simulink model "LQ_observer_simulation"  (R2019a)
settings: Solver=VariableStepAuto  StartTime=0.0  StopTime=24  RelTol=1e-3
values from neighbouring files (symbols this model uses):
  A = modeld.a    [LQR_initialization.m]    (also in LQ_observer_initialization.m; MPC_initialization.m = sysd.a; MagnetoShield_LQ_Initialization.m; MagnetoShield_PolePlacement_Initialization.m)
  B = modeld.b    [LQR_initialization.m]    (also in LQ_observer_initialization.m; MPC_initialization.m = sysd.b; MagnetoShield_LQ_Initialization.m; MagnetoShield_PolePlacement_Initialization.m)
  C = [1 0 0;0 0 1]    [LQR_initialization.m]    (also in LQ_observer_initialization.m = [1 0 0]; MPC_initialization.m = [1 0 0]; MagnetoShield_LQ_Initialization.m; MagnetoShield_PolePlacement_Initialization.m = [1 0 0])
  i0 = 0.00301720799779    [MagnetoShield_Alternative_model.mat]    (also in MagnetoShield_Models_Greybox_SS model.mat = 0.0219057293333)
  K = dlqr(Ai,Bi,Qlq,Rlq)    [LQR_initialization.m]    (also in LQ_observer_initialization.m; MagnetoShield_LQ_Initialization.m; MagnetoShield_PolePlacement_Initialization.m = [0 0 0 1]*inv([Bi Ai*Bi Ai^2*Bi Ai^3*Bi])*phy)
  L = phy*inv([C; C*A; C*A^2])*[0 0 1]'    [LQ_observer_initialization.m]    (also in MagnetoShield_PolePlacement_Initialization.m)
  Ts = 0.001    [LQR_initialization.m]    (also in LQ_observer_initialization.m = 0.002; MPC_initialization.m; MagnetoShield_LQ_Initialization.m = 0.0015; MagnetoShield_PolePlacement_Initialization.m = 0.0015)
  u0 = 0.633613679536    [MagnetoShield_Alternative_model.mat]    (also in MagnetoShield_Models_Greybox_SS model.mat = 4.62338933333)
  y0 = 0.012    [MagnetoShield_Alternative_model.mat]    (also in MagnetoShield_Models_Greybox_SS model.mat = 0.0143094466667)
undefined symbols (not defined in the file or in its folder): DiscIntNeverNeededParam
libraries: simulink x2
settings Model: Creator=jakub  LastModifiedBy=jakub
settings SolverCC: AlgebraicLoopSolver=LineSearch

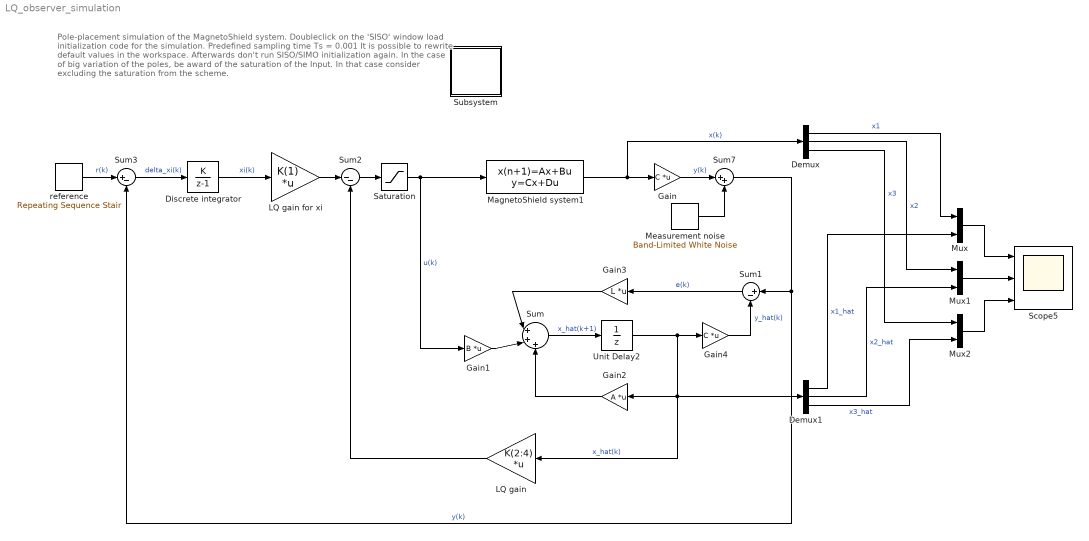
== system LQ_observer_simulation ==
  note: Pole-placement simulation of the  MagnetoShield system.
      | Doubleclick on the 'SISO' window load initialization code for the simulation.
      | Predefined sampling time Ts = 0.001
      | It is possible to rewrite default values in the workspace.  Afterwards don't run SISO/SIMO
      | initialization again.
      |
      | In the case of big variation of the poles, be award of the saturation of the Input. In that case
      | consider excluding the saturation from the scheme.
  Demux : Demux  Outputs=3
  Demux1 : Demux  Outputs=3
  Discrete integrator : DiscreteIntegrator  IntegratorMethod=Accumulation: Forward Euler  SampleTime=Ts  LimitOutput=on  UpperSaturationLimit=1  LowerSaturationLimit=-1  ICPrevOutput=DiscIntNeverNeededParam  ICPrevScaledInput=DiscIntNeverNeededParam
  Gain : Gain  Gain=C  Multiplication=Matrix(K*u)
  Gain1 : Gain  Gain=B  Multiplication=Matrix(K*u)
  Gain2 : Gain  Gain=A  Multiplication=Matrix(K*u)
  Gain3 : Gain  Gain=L  Multiplication=Matrix(K*u)
  Gain4 : Gain  Gain=C  Multiplication=Matrix(K*u)
  LQ gain : Gain  Gain=K(2:4)  Multiplication=Matrix(K*u)
  LQ gain for xi : Gain  Gain=K(1)  Multiplication=Matrix(K*u)
  MagnetoShield system1 : DiscreteStateSpace  A=A  B=B  C=[1 0 0;0 1 0;0 0 1]  D=[0;0;0]  InitialCondition=[0.017-y0;0;0-i0]  SampleTime=Ts
  Measurement noise : simulink/Sources/Band-Limited White Noise  Cov=[(2*10^(-8))^2]  Ts=2*Ts  seed=[23341]
  Mux : Mux  Inputs=2
  Mux1 : Mux  Inputs=2
  Mux2 : Mux  Inputs=2
  Saturation : Saturate  UpperLimit=12-u0  LowerLimit=0-u0
  Scope5 : Scope  NumInputPorts=3
  Subsystem : Subsystem
      settings: OpenFcn=|
      | clear;close all;clc;
      | load '../../../matlab/examples/MagnetoShield/MagnetoShield_Models_Greybox_SS';
      | %% MagnetoShield - Pole-placement simulation and control initialization for Simulink
      | Ts = 0.001;                   % Sampling of the Simulink simulation
      | 
      | % Matrices extraction from model
      | modeld=c2d(model,Ts);           % Discretized linear state-space model
      | A = modeld.a;                   % Extract A
      | B = modeld.b;                   % Extract B
      | C = [1 0 0];                   % Position is measured for integrator 'xi' computation
      | 
      | % Discrete augmented model with integrator state - unstable, unobservable
      | Ai = [1 -C;
      |       zeros(3,1) A];
      | Bi = [0;B];
      | 
      | % Observer gain L computation
      | polesL = [-0.003 0.0006715 -0.00003715]; % desired poles of observer
      | p = poly(polesL);                        % polynomial coeficients
      | I = eye(size(A));
      | phy = p(4)*I+p(3)*A+p(2)*A^2+A^3;
      | L = phy*inv([C; C*A; C*A^2])*[0 0 1]';   % Ackermann's formula for observer
      | 
      | % Pole-placement gain K for augmented system
      | polesK = [0.985 0.5353 0.826 0.9581];       % desired poles of the system
      | p = poly(polesK);                           % polynomial coeficients
      | I = eye(size(Ai));
      | phy = p(5)*I+p(4)*Ai+p(3)*Ai^2+p(2)*Ai^3+Ai^4;
      | K = [0 0 0 1]*inv([Bi Ai*Bi Ai^2*Bi Ai^3*Bi])*phy; % Ackermann's formula for gain K
      mask Display: disp('SISO')
  Sum : Sum  Inputs=|+++
  Sum1 : Sum  Inputs=|+-
  Sum2 : Sum  Inputs=|--
  Sum3 : Sum  Inputs=|+-
  Sum7 : Sum  Inputs=|++
  Unit Delay2 : UnitDelay  InitialCondition=[0.017-y0;0;0-i0]  SampleTime=-1  HasFrameUpgradeWarning=on
  reference : simulink/Sources/Repeating Sequence Stair  OutValues=[ones(1,2000)*(0.013-y0) ones(1,2000)*(0.016-y0) ones(1,2000)*(0.012-y0)].'  tsamp=Ts  OutMin=[]  OutMax=[]  OutDataTypeStr=double  OutputDataTypeScalingMode=double  OutDataType=fixdt(0,8)  ConRadixGroup=Best Precision: Vector-wise  OutScaling=2^-12
  wires:
  Saturation/1 -> MagnetoShield system1/1, Gain1/1  "u(k)"
  Sum2/1 -> Saturation/1
  Discrete integrator/1 -> LQ gain for xi/1  "xi(k)"
  Sum3/1 -> Discrete integrator/1  "delta_xi(k)"
  LQ gain for xi/1 -> Sum2/1
  reference/1 -> Sum3/1  "r(k)"
  LQ gain/1 -> Sum2/2
  MagnetoShield system1/1 -> Demux/1, Gain/1  "x(k)"
  Gain1/1 -> Sum/2
  Unit Delay2/1 -> Gain4/1, Demux1/1, Gain2/1, LQ gain/1  "x_hat(k)"
  Gain2/1 -> Sum/3
  Sum1/1 -> Gain3/1  "e(k)"
  Gain4/1 -> Sum1/2  "y_hat(k)"
  Gain3/1 -> Sum/1
  Sum/1 -> Unit Delay2/1  "x_hat(k+1)"
  Sum7/1 -> Sum1/1, Sum3/2  "y(k)"
  Measurement noise/1 -> Sum7/2
  Gain/1 -> Sum7/1  "y(k)"
  Mux/1 -> Scope5/1
  Mux1/1 -> Scope5/2
  Mux2/1 -> Scope5/3
  Demux/1 -> Mux/1  "x1"
  Demux1/1 -> Mux/2  "x1_hat"
  Demux/2 -> Mux1/1  "x2"
  Demux1/2 -> Mux1/2  "x2_hat"
  Demux1/3 -> Mux2/2  "x3_hat"
  Demux/3 -> Mux2/1  "x3"

== system LQ_observer_simulation/Subsystem ==
